simulink model "Lab2P1"  (R2021b)
settings: Solver=VariableStepAuto  StartTime=0.0  StopTime=40  RelTol=1e-7
libraries: simulink x3
settings Model: Creator=Ahmad  LastModifiedBy=Ahmad

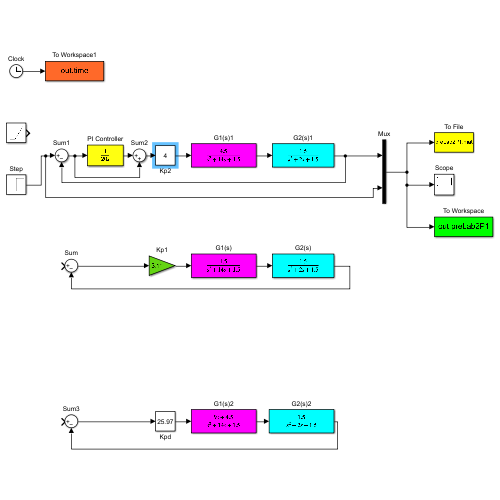
[thumbnail: Simulink's stored preview of the top-level diagram]
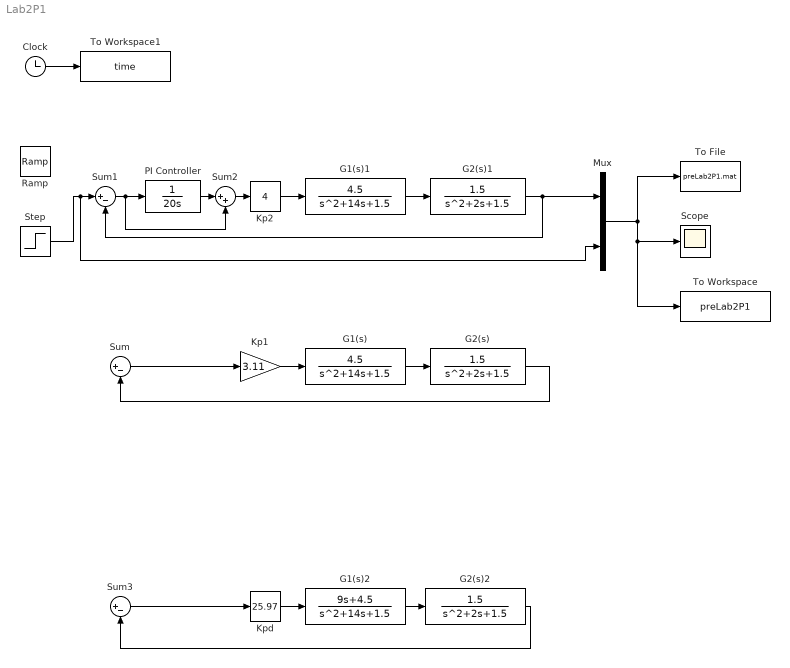
== system Lab2P1 ==
  Clock : Clock
  G1(s) : TransferFcn  Numerator=[4.5]  Denominator=[1 14 1.5]
  G1(s)1 : TransferFcn  Numerator=[4.5]  Denominator=[1 14 1.5]
  G1(s)2 : TransferFcn  Numerator=[9 4.5]  Denominator=[1 14 1.5]
  G2(s) : TransferFcn  Numerator=1.5  Denominator=[1 2 1.5]
  G2(s)1 : TransferFcn  Numerator=[1.5]  Denominator=[1 2 1.5]
  G2(s)2 : TransferFcn  Numerator=[1.5]  Denominator=[1 2 1.5]
  Kp1 : Gain  Gain=3.11
  Kp2 : simulink/Math Operations/Slider Gain  gain=4  low=4  high=10
  Kpd : simulink/Math Operations/Slider Gain  gain=25.97  low=1  high=30
  Mux : Mux  Inputs=2
  PI Controller : TransferFcn  Denominator=[20 0]
  Ramp : simulink/Sources/Ramp  slope=1  start=0  InitialOutput=0
  Scope : Scope
  Step : Step  Time=0  SampleTime=0
  Sum : Sum  Inputs=|+-
  Sum1 : Sum  Inputs=|+-
  Sum2 : Sum  Inputs=|++
  Sum3 : Sum  Inputs=|+-
  To File : ToFile  Filename=preLab2P1.mat  MatrixName=out
  To Workspace : ToWorkspace  VariableName=preLab2P1  SampleTime=-1
  To Workspace1 : ToWorkspace  VariableName=time  SampleTime=-1
  wires:
  Sum/1 -> Kp1/1
  Kp1/1 -> G1(s)/1
  G1(s)/1 -> G2(s)/1
  G2(s)/1 -> Sum/2
  Clock/1 -> To Workspace1/1
  Sum2/1 -> Kp2/1
  PI Controller/1 -> Sum2/1
  Kp2/1 -> G1(s)1/1
  Sum1/1 -> Sum2/2, PI Controller/1
  G1(s)1/1 -> G2(s)1/1
  Sum3/1 -> Kpd/1
  Kpd/1 -> G1(s)2/1
  G1(s)2/1 -> G2(s)2/1
  Mux/1 -> To Workspace/1, Scope/1, To File/1
  G2(s)1/1 -> Mux/1, Sum1/2
  G2(s)2/1 -> Sum3/2
  Step/1 -> Mux/2, Sum1/1
